simulink model "Eq7_8_k1k2k3Linearization"  (R2022b)
settings: Solver=VariableStepAuto  StartTime=0.0  StopTime=10.0  RelTol=1e-3
settings Model: Creator=umber  LastModifiedBy=umber

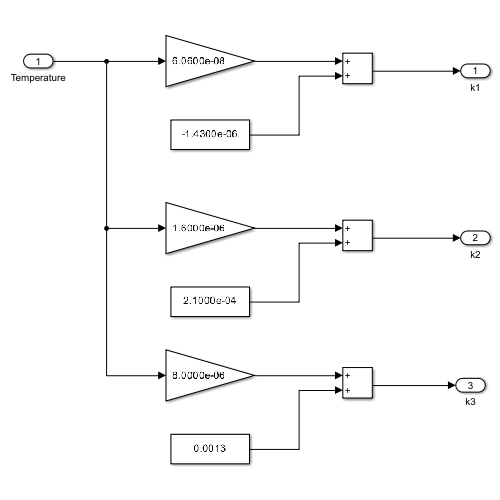
[thumbnail: Simulink's stored preview of the top-level diagram]
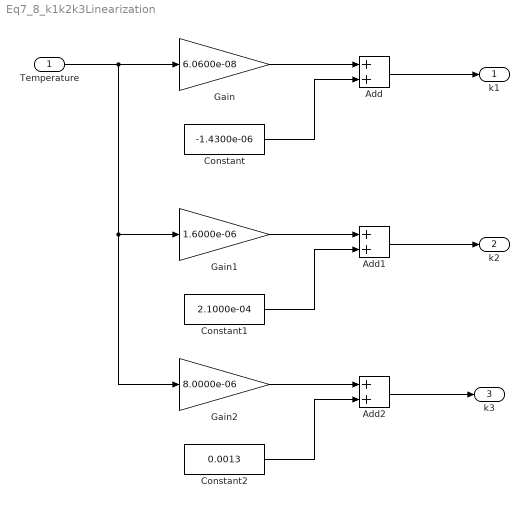
== system Eq7_8_k1k2k3Linearization ==
  Temperature : Inport
  Add : Sum
  Add1 : Sum
  Add2 : Sum
  Constant : Constant  Value=-1.4300e-06
  Constant1 : Constant  Value=2.1000e-04
  Constant2 : Constant  Value=0.0013
  Gain : Gain  Gain=6.0600e-08
  Gain1 : Gain  Gain=1.6000e-06
  Gain2 : Gain  Gain=8.0000e-06
  k1 : Outport
  k2 : Outport  Port=2
  k3 : Outport  Port=3
  wires:
  Gain/1 -> Add/1
  Constant/1 -> Add/2
  Add/1 -> k1/1
  Constant1/1 -> Add1/2
  Gain1/1 -> Add1/1
  Add1/1 -> k2/1
  Temperature/1 -> Gain2/1, Gain1/1, Gain/1
  Gain2/1 -> Add2/1
  Add2/1 -> k3/1
  Constant2/1 -> Add2/2
